simulink model "RedCrane_kinematic_model_joystic"  (R2024a)
settings: Solver=FixedStepAuto  StartTime=0.0  StopTime=inf  FixedStep=Ts  MaxStep=0.005  RelTol=1e-3
values from neighbouring files (symbols this model uses):
  Cartesian_home = [3.55, 0.4, 1.6]'    [enviroment_setup.m]
  M = [1, 0, 0, (L5 + L4 - L1) ... (first row only)    [enviroment_setup.m]
  SList = [ws_mat ... (first row only)    [enviroment_setup.m]
  telescope0 = 0    [enviroment_setup.m]
  thetaList0 = [0, 0,-pi/8, 0, 0]'    [enviroment_setup.m]
  Ts = 0.001    [enviroment_setup.m]
undefined symbols (not defined in the file or in its folder): dp_k_angle_to_stroke, dp_m_angle_to_stroke, p_k_angle_to_stroke, p_k_stroke_to_angle, p_m_angle_to_stroke, p_m_stroke_to_angle, X, Y, Z
libraries: sm_lib x82, nesl_utility x19, fl_lib x16, TcSimInterface x2
(part 1 of 3)
settings Model: Creator=sindr  LastModifiedBy=larso
settings RTWCC: GPUComputeCapability=3.5
settings ConfigComp: PLC_OutputDir=plc_export\FB_JoystickIntegrator  PLC_TargetIDE=twincat3  PLC_MultiTBSigbuilderTimeRange=off  PLC_FoldFBCallOutputVar=off  PLC_RemoveUnusedSSMethodCallArguments=off  PLC_UseCallOutputArgSyntax=off  PLC_EnableUnsignedAndDoubleTypes=off  PLC_EnableUDTSplitting=off  PLC_MaxFieldsInUDT=500  PLC_InlineEnumCastFunction=off

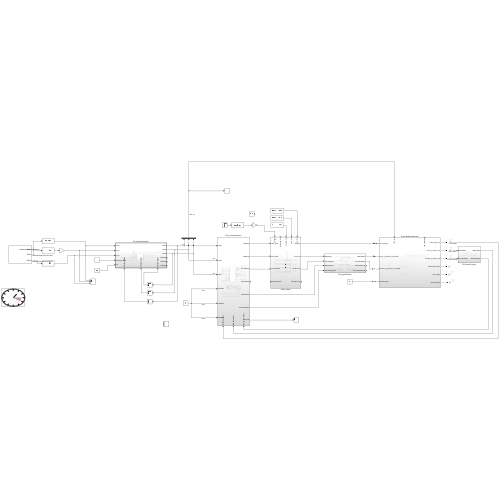
[thumbnail: Simulink's stored preview of the top-level diagram]
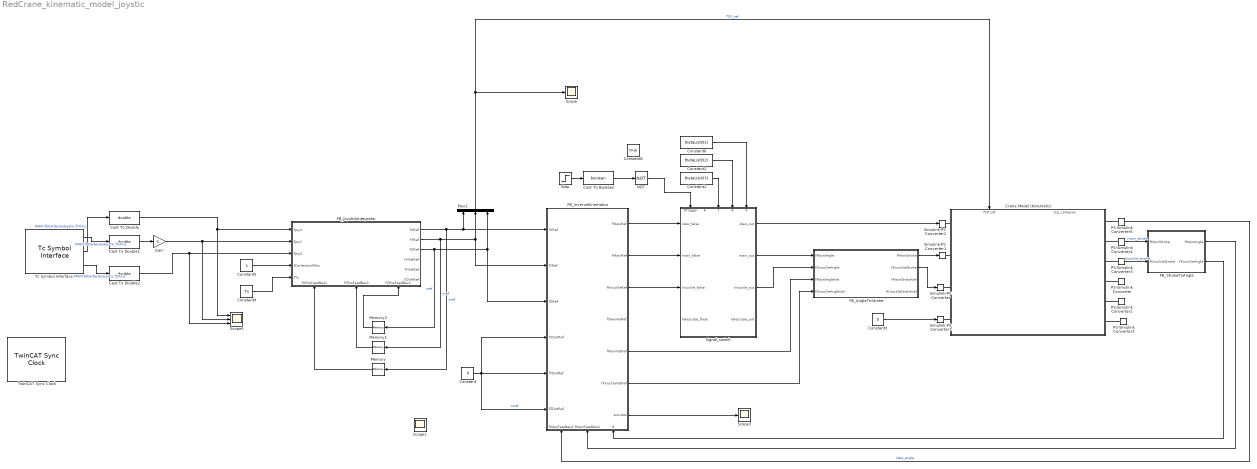
== system RedCrane_kinematic_model_joystic ==
  Cast To Boolean : DataTypeConversion  OutDataTypeStr=boolean  SaturateOnIntegerOverflow=off  RndMeth=Floor
  Cast To Double : DataTypeConversion  OutDataTypeStr=double  SaturateOnIntegerOverflow=off  RndMeth=Floor
  Cast To Double1 : DataTypeConversion  OutDataTypeStr=double  SaturateOnIntegerOverflow=off  RndMeth=Floor
  Cast To Double2 : DataTypeConversion  OutDataTypeStr=double  SaturateOnIntegerOverflow=off  RndMeth=Floor
  Constant : Constant  Value=0
  Constant1 : Constant  Value=thetaList0(3)
  Constant2 : Constant  Value=thetaList0(2)
  Constant3 : Constant  Value=0
  Constant4 : Constant  Value=Ts
  Constant5 : Constant
  Constant6 : Constant  Value=thetaList0(1)
  Constant8 : Constant  Value=true
  Crane Model (Kinematic) : Subsystem
      settings: PortSchema="{\"entries\":[{\"content\":{\"sides\":[{\"content\":{\"connectorIds\":[\"LConn1\",\"LConn2\",\"LConn3\",\"LConn4\"]},\"type\":\"ConnectorPlacement.EquallySpacedRectSide\",\"uuid\":\"4a665765-5f1a-426d-91c2-f3af20fe3627\"},{\"content\":{\"connectorIds\":[\"RConn1\",\"RConn2\",\"RConn3\",\"RConn4\",\"RConn5\",\"RConn6\"],\"side\":\"RIGHT\"},\"type\":\"ConnectorPlacement.EquallySpacedRectSide\",\"uuid\":\"cf43645c-9a50-4bc9-b355-f38e72b1430d\"},{\"content\":{\"connectorIds\":[\"In1\",\"Out1\"],\"side\":\"TOP\"},\"type\":\"ConnectorPlacement.EquallySpacedRectSide\",\"uuid\":\"253dbb23-7a12-4bfe-bf07-7d8403188f09\"}]},\"type\":\"ConnectorPlacement.EquallySpacedConnector\",\"uuid\":\"5ffb1dcc-76b9-4b5c-ba8f-4653fe2f07c9\"}],\"packageUris\":[\"http://schema.mathworks.com/mf0/Connector/R2020b\"],\"version\":\"1.0\"}"
  FB_AngleToStroke : Subsystem
  FB_InverceKinematics : Subsystem
      settings: PortSchema="{\"entries\":[{\"content\":{\"sides\":[{\"content\":{\"connectorIds\":[\"In1\",\"In2\",\"In3\",\"In4\",\"In5\",\"In6\"]},\"type\":\"ConnectorPlacement.EquallySpacedRectSide\",\"uuid\":\"b7f3f39a-cc1b-4519-b948-004466b4d293\"},{\"content\":{\"connectorIds\":[\"Out1\",\"Out2\",\"Out3\",\"Out4\",\"Out5\",\"Out6\",\"Out7\"],\"side\":\"RIGHT\"},\"type\":\"ConnectorPlacement.EquallySpacedRectSide\",\"uuid\":\"cf571c2f-2cc7-4d1d-bbc1-a75d80a0878e\"},{\"content\":{\"side\":\"TOP\"},\"type\":\"ConnectorPlacement.EquallySpacedRectSide\",\"uuid\":\"3f697bd9-7750-4474-8da5-1be48ba53c7e\"},{\"content\":{\"connectorIds\":[\"In7\",\"In8\",\"In9\"],\"side\":\"BOTTOM\"},\"type\":\"ConnectorPlacement.EquallySpacedRectSide\",\"uuid\":\"03fa0a4e-eedb-4a48-8076-446c86a2b4f7\"}]},\"type\":\"ConnectorPlacement.EquallySpacedConnector\",\"uuid\":\"6732c767-80e6-425f-b878-60bd961dd78b\"}],\"packageUris\":[\"http://schema.mathworks.com/mf0/Connector/R2020b\"],\"version\":\"1.0\"}"
  FB_JoystickIntegrator : Subsystem  TreatAsAtomicUnit=on
      settings: PortSchema="{\"entries\":[{\"content\":{\"sides\":[{\"content\":{\"connectorIds\":[\"In1\",\"In2\",\"In3\",\"In4\",\"In5\"]},\"type\":\"ConnectorPlacement.EquallySpacedRectSide\",\"uuid\":\"c5a43198-5d69-4109-b42d-a486a01365c9\"},{\"content\":{\"connectorIds\":[\"Out1\",\"Out2\",\"Out3\",\"Out4\",\"Out5\",\"Out6\"],\"side\":\"RIGHT\"},\"type\":\"ConnectorPlacement.EquallySpacedRectSide\",\"uuid\":\"946526c4-79a3-48b0-aa19-78137d37b9af\"},{\"content\":{\"side\":\"TOP\"},\"type\":\"ConnectorPlacement.EquallySpacedRectSide\",\"uuid\":\"3e7a8b0e-fb34-4723-a326-d25029c5eff4\"},{\"content\":{\"connectorIds\":[\"In6\",\"In7\",\"In8\"],\"side\":\"BOTTOM\"},\"type\":\"ConnectorPlacement.EquallySpacedRectSide\",\"uuid\":\"08712ddf-52dd-443f-9387-c4c8877ba279\"}]},\"type\":\"ConnectorPlacement.EquallySpacedConnector\",\"uuid\":\"e430af44-ed31-458a-a857-840c080c5723\"}],\"packageUris\":[\"http://schema.mathworks.com/mf0/Connector/R2020b\"],\"version\":\"1.0\"}"
  FB_StrokeToAngle : Subsystem
  Gain : Gain  Gain=-1
  Memory : Memory  InitialCondition=Cartesian_home(1)-0.5
  Memory1 : Memory  InitialCondition=Cartesian_home(2)
  Memory2 : Memory  InitialCondition=Cartesian_home(3)
  Mux2 : Mux  Inputs=3
  NOT : Logic  Operator=NOT  IconShape=distinctive  AllPortsSameDT=off  OutDataTypeStr=boolean
  PS-Simulink Converter{,1..5} (6 alike) : nesl_utility/PS-Simulink Converter  PhysicalDomain=network_engine_domain  SubClassName=ps_output  LeftPortType=input  RightPortType=output  PseudoPeriodic=off  Frequencies=[]  VectorFormat=inherit  Unit=inherit  AffineConversion=off
  Scope : Scope
  Scope1 : Scope  NumInputPorts=3
  Scope3 : Scope
  Scope5 : Scope  NumInputPorts=3
  Signal_switch : Subsystem
      settings: PortSchema="{\"entries\":[{\"content\":{\"sides\":[{\"content\":{\"connectorIds\":[\"In1\",\"In2\",\"In3\",\"In4\"]},\"type\":\"ConnectorPlacement.EquallySpacedRectSide\",\"uuid\":\"677999b9-dfe1-4592-affa-fb9b7d257ea0\"},{\"content\":{\"connectorIds\":[\"Out1\",\"Out2\",\"Out3\",\"Out4\"],\"side\":\"RIGHT\"},\"type\":\"ConnectorPlacement.EquallySpacedRectSide\",\"uuid\":\"3f36c443-9717-41bf-801d-3d95a9d66f59\"},{\"content\":{\"connectorIds\":[\"In5\",\"In6\",\"In7\",\"In8\",\"In9\"],\"side\":\"TOP\"},\"type\":\"ConnectorPlacement.EquallySpacedRectSide\",\"uuid\":\"b7ea9b48-8dcd-4abb-ae26-aa1832701a6a\"}]},\"type\":\"ConnectorPlacement.EquallySpacedConnector\",\"uuid\":\"7d55d43f-82cc-482c-a650-cc44ad6cee22\"}],\"packageUris\":[\"http://schema.mathworks.com/mf0/Connector/R2020b\"],\"version\":\"1.0\"}"
  Simulink-PS Converter{,1..3} (4 alike) : nesl_utility/Simulink-PS Converter  PhysicalDomain=network_engine_domain  SubClassName=ps_input  LeftPortType=input  RightPortType=output  PseudoPeriodic=off  Frequencies=[]  NoiseDistribution=none  NoiseParameters=[]  Unit=1  AffineConversion=off  FilteringAndDerivatives=filter  SimscapeFilterOrder=2  InputFilterTimeConstant=0.001  UdotUserProvided=0
  Step : Step  SampleTime=0
  Tc Symbol Interface1 : TcSimInterface/Tc Symbol Interface  ChangeRowColOrder=on  TraceMode=3  DirectFeedThrough=0  SignalLabels=3  PortLabels=2  ExpandBusObjDepth=on  RuntimeConfig=|  SymbolInterfaceInfo=|  SyncClockMode=1
      RuntimeConfig=|
      | <?xml version="1.0" encoding="UTF-8" standalone="no"?>
      | <TcRuntimAdapterProject>
      | 	<DataTypes>
      | 		<DataType>
      | 			<Name GUID="{3BC82419-4CB4-48F5-8384-E3D86DEA2DAE}" Namespace="TcDataExchange">ITcStreamAdsRequestHandler</Name>
      | 			<BitSize X64="64">32</BitSize>
      | 			<BaseType GUID="{00000001-0000-0000-E000-000000000064}">ITcUnknown</BaseType>
      | 			<Method>
      | 				<Name>Send</Name>
      | 				<ReturnType GUID="{18071995-0000-0000-0000-000000000019}">HRESULT</ReturnType>
      | 				<ReturnBitSize>32</ReturnBitSize>
      | 				<Parameter>
      | 					<Name>timeoutMs</Name>
      | 					<Type GUID="{18071995-0000-0000-0000-000000000006}" Optional="1000">INT</Type>
      | 					<BitSize>16</BitSize>
      | 				</Parameter>
      | 				<Parameter>
      | 					<Name>timeStamp</Name>
      | 					<Type GUID="{18071995-0000-0000-0000-00000000000C}" Optional="0">LINT</Type>
      | 					<BitSize>64</BitSize>
      | 				</Parameter>
      | 			</Method>
      | 			<Method>
      | 				<Name>GetResult</Name>
      | 				<ReturnType GUID="{18071995-0000-0000-0000-000000000019}">HRESULT</ReturnType>
      | 				<ReturnBitSize>32</ReturnBitSize>
      | 				<Parameter>
      | 					<Name>pErrorCode</Name>
      | 					<Type GUID="{18071995-0000-0000-0000-000000000009}" PointerTo="1" RpcDirection="out">DINT</Type>
      | 					<BitSize X64="64">32</BitSize>
      | 				</Parameter>
      | 				<Parameter>
      | 					<Name>wait</Name>
      | 					<Type GUID="{18071995-0000-0000-0000-000000000030}" Optional="0">BOOL</Type>
      | 					<BitSize>8</BitSize>
      | 				</Parameter>
      | 			</Method>
      | 			<Method>
      | 				<Name>Cancel</Name>
      | 				<ReturnType GUID="{18071995-0000-0000-0000-000000000019}">HRESULT</ReturnType>
      | 				<ReturnBitSize>32</ReturnBitSize>
      | 			</Method>
      | 			<Hides>
      | 				<Hide GUID="{D5D4EABE-5709-4F1D-A52D-DD780CF3BEE8}"/>
      | 				<Hide GUID="{96230612-048D-4927-9A3E-E69B743416F7}"/>
      | 				<Hide GUID="{F0F623C7-A650-457C-A27C-87DC2B08989E}"/>
      | 				<Hide GUID="{18FCA6B6-AFA6-45DD-BC02-F3037EA03FB7}"/>
      | 				<Hide GUID="{12AC5FFF-B3F6-4F3E-8EDD-8044D44F084F}"/>
      | 				<Hide GUID="{6CDF8435-1307-4137-94DE-D793A77839C3}"/>
      | 				<Hide GUID="{D7B34C9A-90C5-4E79-A290-017678319005}"/>
      | 			</Hides>
      | 		</DataType>
      | 		<DataType>
      | 			<Name GUID="{18071995-0000-0000-0000-000000000041}" TcBaseType="true" HideSubItems="true" CName="AmsNetId">AMSNETID</Name>
      | 			<BitSize>48</BitSize>
      | 			<BaseType GUID="{18071995-0000-0000-0000-000000000001}">BYTE</BaseType>
      | 			<ArrayInfo>
      | 				<LBound>0</LBound>
      | 				<Elements>6</Elements>
      | 			</ArrayInfo>
      | 			<Format>
      | 				<Printf>%d.%d.%d.%d.%d.%d</Printf>
      | 				<Parameter>[0]</Parameter>
      | 				<Parameter>[1]</Parameter>
      | 				<Parameter>[2]</Parameter>
      | 				<Parameter>[3]</Parameter>
      | 				<Parameter>[4]</Parameter>
      | 				<Parameter>[5]</Parameter>
      | 			</Format>
      | 		</DataType>
      | 		<DataType>
      | 			<Name GUID="{18071995-0000-0000-0000-000000000042}" TcBaseType="true" CName="AmsAddr">AMSADDR</Name>
      | 			<BitSize>64</BitSize>
      | 			<SubItem>
      | 				<Name>netId</Name>
      | 				<Type GUID="{18071995-0000-0000-0000-000000000041}">AMSNETID</Type>
      | 				<BitSize>48</BitSize>
      | 				<BitOffs>0</BitOffs>
      | 			</SubItem>
      | 			<SubItem>
      | 				<Name>port</Name>
      | 				<Type GUID="{18071995-0000-0000-0000-000000000004}">WORD</Type>
      | 				<BitSize>16</BitSize>
      | 				<BitOffs>48</BitOffs>
      | 			</SubItem>
      | 			<Format>
      | 				<Printf>%d.%d.%d.%d.%d.%d:%d</Printf>
      | 				<Parameter>.netId[0]</Parameter>
      | 				<Parameter>.netId[1]</Parameter>
      | 				<Parameter>.netId[2]</Parameter>
      | 				<Parameter>.netId[3]</Parameter>
      | 				<Parameter>.netId[4]</Parameter>
      | 				<Parameter>.netId[5]</Parameter>
      | 				<Parameter>.port</Parameter>
      | 			</Format>
      | 			<Format Name="Iec">
      | 				<Printf>(netId:=[%d.%d.%d.%d.%d.%d], port :=%d)</Printf>
      | 				<Parameter>.netId[0]</Parameter>
      | 				<Parameter>.netId[1]</Parameter>
      | 				<Parameter>.netId[2]</Parameter>
      | 				<Parameter>.netId[3]</Parameter>
      | 				<Parameter>.netId[4]</Parameter>
      | 				<Parameter>.netId[5]</Parameter>
      | 				<Parameter>.port</Parameter>
      | 			</Format>
      | 		</DataType>
      | 		<DataType>
      | 			<Name GUID="{EA8975F7-A358-4090-8A68-57EC94D47710}" Namespace="TcDataExchange">SampleCopyInfo</Name>
      | 			<BitSize X64="192">160</BitSize>
      | 			<SubItem>
      | 				<Name>PData</Name>
      | 				<Type GUID="{18071995-0000-0000-0000-000000000001}" PointerTo="1">BYTE</Type>
      | 				<BitSize X64="64">32</BitSize>
      | 				<BitOffs>0</BitOffs>
      | 			</SubItem>
      | 			<SubItem>
      | 				<Name>CbData</Name>
      | 				<Type GUID="{18071995-0000-0000-0000-000000000008}">UDINT</Type>
      | 				<BitSize>32</BitSize>
      | 				<BitOffs X64="64">32</BitOffs>
      | 			</SubItem>
      | 			<SubItem>
      | 				<Name>ErrorCode</Name>
      | 				<Type GUID="{18071995-0000-0000-0000-000000000009}">DINT</Type>
      | 				<BitSize>32</BitSize>
      | 				<BitOffs X64="96">64</BitOffs>
      | 			</SubItem>
      | 			<SubItem>
      | 				<Name>Timestamp</Name>
      | 				<Type GUID="{18071995-0000-0000-0000-00000000000C}">LINT</Type>
      | 				<BitSize>64</BitSize>
      | 				<BitOffs X64="128">96</BitOffs>
      | 			</SubItem>
      | 			<Hides>
      | 				<Hide GUID="{97351DCE-1E32-4BD2-BF27-53E71AD5C45D}"/>
      | 				<Hide GUID="{ED3F58EE-1A95-40F4-94DA-D825E6682038}"/>
      | 				<Hide GUID="{82197966-3CEC-4E84-8982-F64641125942}"/>
      | 			</Hides>
      | 		</DataType>
      | 		<DataType>
      | 			<Name GUID="{9165C8A1-78D1-4B81-89D0-BA48F61AF93B}" Namespace="TcDataExchange">ITcStreamSynchronizer</Name>
      | 			<Comment TxtId=""><![CDATA[Provides time synchronisation between data sources and data sinks in different time contexts. A time context might be a real time TwinCAT system the simulation time of a simulation tool or the basic time stamp of logged data in a database.]]></Comment>
      | 			<BitSize X64="64">32</BitSize>
      | 			<BaseType GUID="{00000001-0000-0000-E000-000000000064}">ITcUnknown</BaseType>
      | 			<Method>
      | 				<Name>RegisterTimeContext</Name>
      | 				<Comment><![CDATA[Registers a time context for synchronization. Registration has to be completet for all time contexts before starting the communication. ]]></Comment>
      | 				<ReturnType GUID="{18071995-0000-0000-0000-000000000019}">HRESULT</ReturnType>
      | 				<ReturnBitSize>32</ReturnBitSize>
      | 				<Parameter>
      | 					<Name>pSyncId</Name>
      | 					<Comment><![CDATA[Unique identifier of the time context. This might be e.g. the AmsNetId of a TwinCAT system or a ULINT representation of a logged dataset.]]></Comment>
      | 					<Type GUID="{18071995-0000-0000-0000-000000000021}" PointerTo="1">GUID</Type>
      | 					<BitSize X64="64">32</BitSize>
      | 				</Parameter>
      | 				<Parameter>
      | 					<Name>timeStamp</Name>
      | 					<Comment><![CDATA[Timestamp of the first received sample]]></Comment>
      | 					<Type GUID="{18071995-0000-0000-0000-00000000000C}">LINT</Type>
      | 					<BitSize>64</BitSize>
      | 				</Parameter>
      | 			</Method>
      | 			<Method>
      | 				<Name>TransformTime</Name>
      | 				<ReturnType GUID="{18071995-0000-0000-0000-000000000019}">HRESULT</ReturnType>
      | 				<ReturnBitSize>32</ReturnBitSize>
      | 				<Parameter>
      | 					<Name>pSourceSyncId</Name>
      | 					<Comment><![CDATA[Unique identifier of the source time context.]]></Comment>
      | 					<Type GUID="{18071995-0000-0000-0000-000000000021}" PointerTo="1">GUID</Type>
      | 					<BitSize X64="64">32</BitSize>
      | 				</Parameter>
      | 				<Parameter>
      | 					<Name>pSinkSyncId</Name>
      | 					<Comment><![CDATA[Unique identifier of the sink time context.]]></Comment>
      | 					<Type GUID="{18071995-0000-0000-0000-000000000021}" PointerTo="1">GUID</Type>
      | 					<BitSize X64="64">32</BitSize>
      | 				</Parameter>
      | 				<Parameter>
      | 					<Name>timeStamp</Name>
      | 					<Comment><![CDATA[Expects the sink timestamp and returns the appropriate source timestamp.
      | If the specified sink sync ID is unknown, the sink timestamp is register as its start time.]]></Comment>
      | 					<Type GUID="{18071995-0000-0000-0000-00000000000C}" ReferenceTo="true">LINT</Type>
      | 					<BitSize X64="64">32</BitSize>
      | 				</Parameter>
      | 			</Method>
      | 			<Hides>
      | 				<Hide GUID="{92EEAEA2-3DA4-48E7-A741-8C78A0326B08}"/>
      | 				<Hide GUID="{4F229E80-CBB0-4042-863E-770932FFF733}"/>
      | 				<Hide GUID="{BDB7FF6F-6144-4421-92B4-18BEEF6031E5}"/>
      | 				<Hide GUID="{5983EBFA-553B-4573-BA8B-8294D34A7664}"/>
      | 				<Hide GUID="{8DB2BF24-3BB5-46A0-91E8-A1C18BBD84A4}"/>
      | 				<Hide GUID="{865BE9CA-A112-4D69-9BA4-637F3C45508E}"/>
      | 				<Hide GUID="{5732FA65-993E-4C75-A424-0F55737580DD}"/>
      | 				<Hide GUID="{E7473B34-EFDE-47D8-AEF4-4BDF09E5E870}"/>
      | 				<Hide GUID="{BA2BDE8E-989A-4914-98EA-E301FA5E0803}"/>
      | 				<Hide GUID="{59CDFCE5-FBBF-47C8-A338-68414C56327E}"/>
      | 				<Hide GUID="{0C52276D-0720-4AEF-8258-67851E35C9C8}"/>
      | 				<Hide GUID="{4A5DD8C7-96C5-4D47-A240-8E493B9287A7}"/>
      | 			</Hides>
      | 		</DataType>
      | 		<DataType>
      | 			<Name GUID="{CD026BE9-DD1E-4238-B09F-CDE426934EFB}" Namespace="TcDataExchange">ITcStreamSyncDataSink</Name>
      | 			<BitSize X64="64">32</BitSize>
      | 			<BaseType GUID="{00000001-0000-0000-E000-000000000064}">ITcUnknown</BaseType>
      | 			<Method>
      | 				<Name>WriteSamples</Name>
      | 				<ReturnType GUID="{18071995-0000-0000-0000-000000000019}">HRESULT</ReturnType>
      | 				<ReturnBitSize>32</ReturnBitSize>
      | 				<Parameter>
      | 					<Name>writerOid</Name>
      | 					<Type GUID="{18071995-0000-0000-0000-00000000000F}">OTCID</Type>
      | 					<BitSize>32</BitSize>
      | 				</Parameter>
      | 				<Parameter>
      | 					<Name>pSyncId</Name>
      | 					<Comment><![CDATA[Unique identifier of the time context. This might be e.g. the AmsNetId of a TwinCAT system or a ULINT representation of a logged dataset.]]></Comment>
      | 					<Type GUID="{18071995-0000-0000-0000-000000000021}" PointerTo="1" RpcDirection="in">GUID</Type>
      | 					<BitSize X64="64">32</BitSize>
      | 				</Parameter>
      | 				<Parameter>
      | 					<Name>sampleSize</Name>
      | 					<Type GUID="{18071995-0000-0000-0000-000000000008}" RpcDirection="in">UDINT</Type>
      | 					<BitSize>32</BitSize>
      | 				</Parameter>
      | 				<Parameter>
      | 					<Name>sampleCount</Name>
      | 					<Type GUID="{18071995-0000-0000-0000-000000000008}" RpcDirection="in">UDINT</Type>
      | 					<BitSize>32</BitSize>
      | 				</Parameter>
      | 				<Parameter>
      | 					<Name>pSamples</Name>
      | 					<Type GUID="{18071995-0000-0000-0000-000000000001}" PointerTo="1" RpcDirection="in">BYTE</Type>
      | 					<BitSize X64="64">32</BitSize>
      | 				</Parameter>
      | 				<Parameter>
      | 					<Name>pErrorCodes</Name>
      | 					<Type GUID="{18071995-0000-0000-0000-000000000009}" PointerTo="1" RpcDirection="in" RpcLengthIs="sampleCount" Optional="0">DINT</Type>
      | 					<BitSize X64="64">32</BitSize>
      | 				</Parameter>
      | 				<Parameter>
      | 					<Name>pTimeStamps</Name>
      | 					<Type GUID="{18071995-0000-0000-0000-00000000000C}" PointerTo="1" RpcDirection="in" Optional="0">LINT</Type>
      | 					<BitSize X64="64">32</BitSize>
      | 				</Parameter>
      | 				<Parameter>
      | 					<Name>sampleStride</Name>
      | 					<Type GUID="{18071995-0000-0000-0000-000000000006}" Optional="-1">INT</Type>
      | 					<BitSize>16</BitSize>
      | 				</Parameter>
      | 				<Parameter>
      | 					<Name>errorCodeStride</Name>
      | 					<Type GUID="{18071995-0000-0000-0000-000000000006}" Optional="-1">INT</Type>
      | 					<BitSize>16</BitSize>
      | 				</Parameter>
      | 				<Parameter>
      | 					<Name>timeStampStride</Name>
      | 					<Type GUID="{18071995-0000-0000-0000-000000000006}" Optional="-1">INT</Type>
      | 					<BitSize>16</BitSize>
      | 				</Parameter>
      | 			</Method>
      | 			<Method>
      | 				<Name>WriteSamples</Name>
      | 				<ReturnType GUID="{18071995-0000-0000-0000-000000000019}">HRESULT</ReturnType>
      | 				<ReturnBitSize>32</ReturnBitSize>
      | 				<Parameter>
      | 					<Name>pSyncId</Name>
      | 					<Comment><![CDATA[Unique identifier of the time context. This might be e.g. the AmsNetId of a TwinCAT system or a ULINT representation of a logged dataset.]]></Comment>
      | 					<Type GUID="{18071995-0000-0000-0000-000000000021}" PointerTo="1" RpcDirection="in">GUID</Type>
      | 					<BitSize X64="64">32</BitSize>
      | 				</Parameter>
      | 				<Parameter>
      | 					<Name>sampleCount</Name>
      | 					<Type GUID="{18071995-0000-0000-0000-000000000008}" RpcDirection="in">UDINT</Type>
      | 					<BitSize>32</BitSize>
      | 				</Parameter>
      | 				<Parameter>
      | 					<Name>pSampleCopyInfo</Name>
      | 					<Type GUID="{EA8975F7-A358-4090-8A68-57EC94D47710}" Namespace="TcDataExchange" PointerTo="1" RpcDirection="in">SampleCopyInfo</Type>
      | 					<BitSize X64="64">32</BitSize>
      | 				</Parameter>
      | 			</Method>
      | 			<Method>
      | 				<Name>GetSynchronizer</Name>
      | 				<ReturnType GUID="{18071995-0000-0000-0000-000000000019}">HRESULT</ReturnType>
      | 				<ReturnBitSize>32</ReturnBitSize>
      | 				<Parameter>
      | 					<Name>ppSynchronizer</Name>
      | 					<Type GUID="{9165C8A1-78D1-4B81-89D0-BA48F61AF93B}" Namespace="TcDataExchange" PointerTo="1">ITcStreamSynchronizer</Type>
      | 					<BitSize X64="64">32</BitSize>
      | 				</Parameter>
      | 			</Method>
      | 			<Hides>
      | 				<Hide GUID="{81DCA55F-6320-4831-9AAA-FA43AB137432}"/>
      | 				<Hide GUID="{7F649ADE-4559-4067-8B4B-52A9AFF9D566}"/>
      | 				<Hide GUID="{1ACFD07C-85DE-4584-B8DF-DCE4B2186A56}"/>
      | 				<Hide GUID="{001A190B-B452-4F64-99FE-587E5CB0E1C9}"/>
      | 				<Hide GUID="{D321BA65-82B7-4E6F-9E21-63A2CF6BE6E4}"/>
      | 				<Hide GUID="{59469964-9185-47B0-8E1F-A41A5243C9A7}"/>
      | 				<Hide GUID="{50E978C6-91D0-425B-941B-FF6E10C52E19}"/>
      | 				<Hide GUID="{2B2E9620-3973-41C2-927F-D2660E0236D6}"/>
      | 				<Hide GUID="{4C925035-5840-4BD6-BA08-B62ECBE72975}"/>
      | 				<Hide GUID="{C77882D3-FF3C-4E62-96AB-AB67CC7FA3B0}"/>
      | 				<Hide GUID="{7619FBA7-E9CC-47D7-AEE2-2BAE64602CA0}"/>
      | 				<Hide GUID="{CACC088B-451D-4181-939C-F28316D26AF6}"/>
      | 				<Hide GUID="{1701C290-46E1-4294-AA28-C9384682A3D1}"/>
      | 				<Hide GUID="{D4FE94A8-2959-45FC-B97D-A36FE755F217}"/>
      | 				<Hide GUID="{62A55225-FD8F-4450-A003-5E82394FD0D1}"/>
      | 				<Hide GUID="{7DA0071B-E1EB-4FCF-B5BE-180B5FA4841C}"/>
      | 				<Hide GUID="{D2B3A2BF-4D63-4F61-853F-3333868D1C42}"/>
      | 				<Hide GUID="{C8B9397B-AE09-4B06-8883-D01BD9BBDEFB}"/>
      | 				<Hide GUID="{276A390F-8541-45D2-8A94-8E3B6B609E81}"/>
      | 				<Hide GUID="{F4C49966-BC54-424E-A3C6-69D9FBDDE2BC}"/>
      | 			</Hides>
      | 		</DataType>
      | 		<DataType>
      | 			<Name GUID="{877CB26F-4EC1-469B-9F87-706DDBDA821F}" Namespace="TcDataExchange">ITcStreamSyncDataSource</Name>
      | 			<BitSize X64="64">32</BitSize>
      | 			<BaseType GUID="{00000001-0000-0000-E000-000000000064}">ITcUnknown</BaseType>
      | 			<Method>
      | 				<Name>ReadSamples</Name>
      | 				<ReturnType GUID="{18071995-0000-0000-0000-000000000019}">HRESULT</ReturnType>
      | 				<ReturnBitSize>32</ReturnBitSize>
      | 				<Parameter>
      | 					<Name>readerOid</Name>
      | 					<Type GUID="{18071995-0000-0000-0000-00000000000F}">OTCID</Type>
      | 					<BitSize>32</BitSize>
      | 				</Parameter>
      | 				<Parameter>
      | 					<Name>pSyncId</Name>
      | 					<Comment><![CDATA[Unique identifier of the time context. This might be e.g. the AmsNetId of a TwinCAT system or a ULINT representation of a logged dataset.]]></Comment>
      | 					<Type GUID="{18071995-0000-0000-0000-000000000021}" PointerTo="1" RpcDirection="in">GUID</Type>
      | 					<BitSize X64="64">32</BitSize>
      | 				</Parameter>
      | 				<Parameter>
      | 					<Name>sampleSize</Name>
      | 					<Type GUID="{18071995-0000-0000-0000-000000000008}" RpcDirection="in">UDINT</Type>
      | 					<BitSize>32</BitSize>
      | 				</Parameter>
      | 				<Parameter>
      | 					<Name>sampleCount</Name>
      | 					<Type GUID="{18071995-0000-0000-0000-000000000008}" ReferenceTo="true" RpcDirection="in">UDINT</Type>
      | 					<BitSize X64="64">32</BitSize>
      | 				</Parameter>
      | 				<Parameter>
      | 					<Name>pSamples</Name>
      | 					<Type GUID="{18071995-0000-0000-0000-000000000001}" PointerTo="1" RpcDirection="out">BYTE</Type>
      | 					<BitSize X64="64">32</BitSize>
      | 				</Parameter>
      | 				<Parameter>
      | 					<Name>pErrorCodes</Name>
      | 					<Type GUID="{18071995-0000-0000-0000-000000000009}" PointerTo="1" RpcDirection="out" RpcLengthIs="sampleCount" Optional="0">DINT</Type>
      | 					<BitSize X64="64">32</BitSize>
      | 				</Parameter>
      | 				<Parameter>
      | 					<Name>pTimeStamps</Name>
      | 					<Type GUID="{18071995-0000-0000-0000-00000000000C}" PointerTo="1" RpcDirection="out" RpcLengthIs="sampleCount" Optional="0">LINT</Type>
      | 					<BitSize X64="64">32</BitSize>
      | 				</Parameter>
      | 				<Parameter>
      | 					<Name>timeStamp</Name>
      | 					<Type GUID="{18071995-0000-0000-0000-00000000000C}" Optional="0">LINT</Type>
      | 					<BitSize>64</BitSize>
      | 				</Parameter>
      | 				<Parameter>
      | 					<Name>nextTimeStamp</Name>
      | 					<Type GUID="{18071995-0000-0000-0000-00000000000C}" Optional="0">LINT</Type>
      | 					<BitSize>64</BitSize>
      | 				</Parameter>
      | 			</Method>
      | 			<Method>
      | 				<Name>ReadSamples</Name>
      | 				<ReturnType GUID="{18071995-0000-0000-0000-000000000019}">HRESULT</ReturnType>
      | 				<ReturnBitSize>32</ReturnBitSize>
      | 				<Parameter>
      | 					<Name>readerOid</Name>
      | 					<Type GUID="{18071995-0000-0000-0000-00000000000F}">OTCID</Type>
      | 					<BitSize>32</BitSize>
      | 				</Parameter>
      | 				<Parameter>
      | 					<Name>pSyncId</Name>
      | 					<Comment><![CDATA[Unique identifier of the time context. This might be e.g. the AmsNetId of a TwinCAT system or a ULINT representation of a logged dataset.]]></Comment>
      | 					<Type GUID="{18071995-0000-0000-0000-000000000021}" PointerTo="1" RpcDirection="in">GUID</Type>
      | 					<BitSize X64="64">32</BitSize>
      | 				</Parameter>
      | 				<Parameter>
      | 					<Name>sampleCount</Name>
      | 					<Type GUID="{18071995-0000-0000-0000-000000000008}" ReferenceTo="true" RpcDirection="in">UDINT</Type>
      | 					<BitSize X64="64">32</BitSize>
      | 				</Parameter>
      | 				<Parameter>
      | 					<Name>pSampleCopyInfo</Name>
      | 					<Type GUID="{EA8975F7-A358-4090-8A68-57EC94D47710}" Namespace="TcDataExchange" PointerTo="1" RpcLengthIs="sampleCount">SampleCopyInfo</Type>
      | 					<BitSize X64="64">32</BitSize>
      | 				</Parameter>
      | 				<Parameter>
      | 					<Name>timeStamp</Name>
      | 					<Type GUID="{18071995-0000-0000-0000-00000000000C}" Optional="0">LINT</Type>
      | 					<BitSize>64</BitSize>
      | 				</Parameter>
      | 				<Parameter>
      | 					<Name>nextTimeStamp</Name>
      | 					<Type GUID="{18071995-0000-0000-0000-00000000000C}" Optional="0">LINT</Type>
      | 					<BitSize>64</BitSize>
      | 				</Parameter>
      | 			</Method>
      | 			<Method>
      | 				<Name>ReadSample</Name>
      | 				<ReturnType GUID="{18071995-0000-0000-0000-000000000019}">HRESULT</ReturnType>
      | 				<ReturnBitSize>32</ReturnBitSize>
      | 				<Parameter>
      | 					<Name>readerOid</Name>
      | 					<Type GUID="{18071995-0000-0000-0000-00000000000F}">OTCID</Type>
      | 					<BitSize>32</BitSize>
      | 				</Parameter>
      | 				<Parameter>
      | 					<Name>pSyncId</Name>
      | 					<Comment><![CDATA[Unique identifier of the time context. This might be e.g. the AmsNetId of a TwinCAT system or a ULINT representation of a logged dataset.]]></Comment>
      | 					<Type GUID="{18071995-0000-0000-0000-000000000021}" PointerTo="1" RpcDirection="in">GUID</Type>
      | 					<BitSize X64="64">32</BitSize>
      | 				</Parameter>
      | 				<Parameter>
      | 					<Name>sampleSize</Name>
      | 					<Type GUID="{18071995-0000-0000-0000-000000000008}" RpcDirection="in">UDINT</Type>
      | 					<BitSize>32</BitSize>
      | 				</Parameter>
      | 				<Parameter>
      | 					<Name>timeStamp</Name>
      | 					<Type GUID="{18071995-0000-0000-0000-00000000000C}" RpcDirection="in">LINT</Type>
      | 					<BitSize>64</BitSize>
      | 				</Parameter>
      | 				<Parameter>
      | 					<Name>pSample</Name>
      | 					<Type GUID="{18071995-0000-0000-0000-000000000001}" PointerTo="1" RpcDirection="out">BYTE</Type>
      | 					<BitSize X64="64">32</BitSize>
      | 				</Parameter>
      | 				<Parameter>
      | 					<Name>nextTimeStamp</Name>
      | 					<Type GUID="{18071995-0000-0000-0000-00000000000C}" Optional="0">LINT</Type>
      | 					<BitSize>64</BitSize>
      | 				</Parameter>
      | 				<Parameter>
      | 					<Name>timeoutMs</Name>
      | 					<Type GUID="{18071995-0000-0000-0000-000000000006}" Optional="0">INT</Type>
      | 					<BitSize>16</BitSize>
      | 				</Parameter>
      | 			</Method>
      | 			<Method>
      | 				<Name>ReportTransferState</Name>
      | 				<ReturnType GUID="{18071995-0000-0000-0000-000000000019}">HRESULT</ReturnType>
      | 				<ReturnBitSize>32</ReturnBitSize>
      | 				<Parameter>
      | 					<Name>sampleCount</Name>
      | 					<Type GUID="{18071995-0000-0000-0000-000000000008}" RpcDirection="in">UDINT</Type>
      | 					<BitSize>32</BitSize>
      | 				</Parameter>
      | 				<Parameter>
      | 					<Name>pTimeStamps</Name>
      | 					<Type GUID="{18071995-0000-0000-0000-00000000000B}" PointerTo="1" RpcDirection="in" RpcLengthIs="sampleCount">ULINT</Type>
      | 					<BitSize X64="64">32</BitSize>
      | 				</Parameter>
      | 				<Parameter>
      | 					<Name>pErrorCodes</Name>
      | 					<Type GUID="{18071995-0000-0000-0000-000000000009}" PointerTo="1" RpcDirection="in" RpcLengthIs="sampleCount">DINT</Type>
      | 					<BitSize X64="64">32</BitSize>
      | 				</Parameter>
      | 			</Method>
      | 			<Hides>
      | 				<Hide GUID="{82F08223-5E24-40E3-9A21-D5759118CBB7}"/>
      | 				<Hide GUID="{BC021C3C-19AB-41D1-A0EC-9FBFBB8814F1}"/>
      | 				<Hide GUID="{50FC6FF1-2968-4C30-A0C6-937238137C4E}"/>
      | 				<Hide GUID="{728E78FA-EADA-4107-BAE9-D37F8F7B9F91}"/>
      | 				<Hide GUID="{C24D9FA7-A6FF-412B-8385-D45B3613DB25}"/>
      | 				<Hide GUID="{57723EE7-8620-4304-9DD4-46EA4C8A93FC}"/>
      | 				<Hide GUID="{F29D82E8-B39D-4DDA-9326-A3CDC9CBBA4B}"/>
      | 				<Hide GUID="{53ABEA21-7053-4CE3-9300-41FAB67AF005}"/>
      | 				<Hide GUID="{E5414156-6DAA-44BD-9EFA-B9044BBB9FAE}"/>
      | 				<Hide GUID="{160EC4BE-B114-439C-A4F5-197C13AE54BE}"/>
      | 				<Hide GUID="{D7DC26B1-9810-47CC-88D8-D4B09543C26B}"/>
      | 				<Hide GUID="{2F3D2A75-7CFD-4B59-86BD-5AB92BFF5C6C}"/>
      | 				<Hide GUID="{205321E8-A331-4955-8C9E-2D60B6EAF5D8}"/>
      | 				<Hide GUID="{BA3232D2-3C23-413B-A027-D772D0C5AA3E}"/>
      | 				<Hide GUID="{FAF64FB6-67DC-4FA2-8863-A3D939045635}"/>
      | 				<Hide GUID="{5DF157ED-EE29-443B-ACD3-F7E4A686CAC8}"/>
      | 				<Hide GUID="{E20D9512-3189-4583-A5D1-6C522392AD43}"/>
      | 				<Hide GUID="{F98C9E94-47EC-40AD-AC60-E0D0FB029194}"/>
      | 				<Hide GUID="{4ED484EC-9FA9-4567-9D83-41D6BB37A214}"/>
      | 				<Hide GUID="{48244BB5-38E0-4EC3-BEA8-67AE38BFA0E5}"/>
      | 				<Hide GUID="{D85B01E0-4969-4DCF-BE5B-BBCBD9E96328}"/>
      | 				<Hide GUID="{DF45952D-9A36-4D45-934F-003F97EE2709}"/>
      | 				<Hide GUID="{582175E1-C08A-4DA1-8055-83DB0709413E}"/>
      | 				<Hide GUID="{292D2B8D-7D29-4791-A738-0FA706E6D7C7}"/>
      | 				<Hide GUID="{9660BF40-2F53-4366-912D-5DA5488BD995}"/>
      | 				<Hide GUID="{AA37253E-123B-4A23-88B2-320766B046C5}"/>
      | 				<Hide GUID="{8A9F48A1-52FB-47FA-AF47-A72CB42C8F27}"/>
      | 				<Hide GUID="{DC5918CB-E382-4038-B2ED-00FF581EA40F}"/>
      | 				<Hide GUID="{754FA08E-4EE5-4772-B861-C4D9514E5FE2}"/>
      | 				<Hide GUID="{2C0F86D1-13AC-46DB-BFB0-A62CF0B8CEE8}"/>
      | 			</Hides>
      | 		</DataType>
      | 		<DataType>
      | 			<Name GUID="{2919D6B4-47C4-4AE8-B706-E94C497ECB99}" Namespace="TcDataExchange">NotificationTransMode</Name>
      | 			<BitSize>16</BitSize>
      | 			<BaseType GUID="{18071995-0000-0000-0000-000000000006}">INT</BaseType>
      | 			<EnumInfo>
      | 				<Text><![CDATA[NoTrans]]></Text>
      | 				<Enum>0</Enum>
      | 			</EnumInfo>
      | 			<EnumInfo>
      | 				<Text><![CDATA[ServerCycle]]></Text>
      | 				<Enum>3</Enum>
      | 			</EnumInfo>
      | 			<EnumInfo>
      | 				<Text><![CDATA[OnChange]]></Text>
      | 				<Enum>4</Enum>
      | 			</EnumInfo>
      | 			<Hides>
      | 				<Hide GUID="{79465139-46B4-43EB-B7FF-967BF64C3367}"/>
      | 				<Hide GUID="{AE2F4BB5-B98E-4C79-AC26-086A9CF7EAC6}"/>
      | 				<Hide GUID="{ECF929B2-79C7-483F-A3DC-06B91AFD531C}"/>
      | 				<Hide GUID="{4E4B27B2-E550-42F1-92B6-1EFABDB0481B}"/>
      | 			</Hides>
      | 		</DataType>
      | 		<DataType>
      | 			<Name GUID="{B75DDCED-7BC8-45F5-8D80-27345642612D}" Namespace="TcDataExchange">NotificationState</Name>
      | 			<BitSize>16</BitSize>
      | 			<BaseType GUID="{18071995-0000-0000-0000-000000000006}">INT</BaseType>
      | 			<EnumInfo>
      | 				<Text><![CDATA[Stop]]></Text>
      | 				<Enum>0</Enum>
      | 			</EnumInfo>
      | 			<EnumInfo>
      | 				<Text><![CDATA[Starting]]></Text>
      | 				<Enum>1</Enum>
      | 			</EnumInfo>
      | 			<EnumInfo>
      | 				<Text><![CDATA[Run]]></Text>
      | 				<Enum>2</Enum>
      | 			</EnumInfo>
      | 			<EnumInfo>
      | 				<Text><![CDATA[Stopping]]></Text>
      | 				<Enum>3</Enum>
      | 			</EnumInfo>
      | 			<EnumInfo>
      | 				<Text><![CDATA[StartError]]></Text>
      | 				<Enum>4</Enum>
      | 			</EnumInfo>
      | 			<EnumInfo>
      | 				<Text><![CDATA[StopError]]></Text>
      | 				<Enum>5</Enum>
      | 			</EnumInfo>
      | 			<Hides>
      | 				<Hide GUID="{BEEA3766-C152-4B4D-80E7-6332297C102B}"/>
      | 			</Hides>
      | 		</DataType>
      | 		<DataType>
      | 			<Name GUID="{BCEA2DD9-BE3C-4A28-A404-258B4399FDEA}" Namespace="TcDataExchange">ITcStreamAdsNotificationHandler</Name>
      | 			<BitSize X64="64">32</BitSize>
      | 			<BaseType GUID="{00000001-0000-0000-E000-000000000064}">ITcUnknown</BaseType>
      | 			<Method>
      | 				<Name>Start</Name>
      | 				<ReturnType GUID="{18071995-0000-0000-0000-000000000019}">HRESULT</ReturnType>
      | 				<ReturnBitSize>32</ReturnBitSize>
      | 				<Parameter>
      | 					<Name>sampleTime100ns</Name>
      | 					<Comment><![CDATA[SampleTime in 100ns. If the value is 0 or too small, the requests will be send as fast as possible.]]></Comment>
      | 					<Type GUID="{18071995-0000-0000-0000-000000000008}" Optional="0">UDINT</Type>
      | 					<BitSize>32</BitSize>
      | 				</Parameter>
      | 				<Parameter>
      | 					<Name>delayTime100ns</Name>
      | 					<Comment><![CDATA[DelayTime in 100ns.]]></Comment>
      | 					<Type GUID="{18071995-0000-0000-0000-000000000008}" Optional="10">UDINT</Type>
      | 					<BitSize>32</BitSize>
      | 				</Parameter>
      | 				<Parameter>
      | 					<Name>createTimeoutMs</Name>
      | 					<Type GUID="{18071995-0000-0000-0000-000000000006}" Optional="1000">INT</Type>
      | 					<BitSize>16</BitSize>
      | 				</Parameter>
      | 				<Parameter>
      | 					<Name>transMode</Name>
      | 					<Type GUID="{2919D6B4-47C4-4AE8-B706-E94C497ECB99}" Namespace="TcDataExchange" Optional="0">NotificationTransMode</Type>
      | 					<BitSize>16</BitSize>
      | 				</Parameter>
      | 			</Method>
      | 			<Method>
      | 				<Name>Stop</Name>
      | 				<ReturnType GUID="{18071995-0000-0000-0000-000000000019}">HRESULT</ReturnType>
      | 				<ReturnBitSize>32</ReturnBitSize>
      | 				<Parameter>
      | 					<Name>stopTimeoutMs</Name>
      | 					<Type GUID="{18071995-0000-0000-0000-000000000006}" Optional="1000">INT</Type>
      | 					<BitSize>16</BitSize>
      | 				</Parameter>
      | 			</Method>
      | 			<Method>
      | 				<Name>GetState</Name>
      | 				<ReturnType GUID="{18071995-0000-0000-0000-000000000019}">HRESULT</ReturnType>
      | 				<ReturnBitSize>32</ReturnBitSize>
      | 				<Parameter>
      | 					<Name>pState</Name>
      | 					<Type GUID="{B75DDCED-7BC8-45F5-8D80-27345642612D}" Namespace="TcDataExchange" PointerTo="1">NotificationState</Type>
      | 					<BitSize X64="64">32</BitSize>
      | 				</Parameter>
      | 				<Parameter>
      | 					<Name>pErrorCode</Name>
      | 					<Type GUID="{18071995-0000-0000-0000-000000000009}" PointerTo="1">DINT</Type>
      | 					<BitSize X64="64">32</BitSize>
      | 				</Parameter>
      | 			</Method>
      | 			<Method>
      | 				<Name>WaitFor</Name>
      | 				<ReturnType GUID="{18071995-0000-0000-0000-000000000019}">HRESULT</ReturnType>
      | 				<ReturnBitSize>32</ReturnBitSize>
      | 				<Parameter>
      | 					<Name>targetState</Name>
      | 					<Type GUID="{B75DDCED-7BC8-45F5-8D80-27345642612D}" Namespace="TcDataExchange">NotificationState</Type>
      | 					<BitSize>16</BitSize>
      | 				</Parameter>
      | 				<Parameter>
      | 					<Name>wait</Name>
      | 					<Type GUID="{18071995-0000-0000-0000-000000000030}" Optional="1">BOOL</Type>
      | 					<BitSize>8</BitSize>
      | 				</Parameter>
      | 			</Method>
      | 			<Method>
      | 				<Name>LastIndicationTime</Name>
      | 				<ReturnType GUID="{18071995-0000-0000-0000-000000000019}">HRESULT</ReturnType>
      | 				<ReturnBitSize>32</ReturnBitSize>
      | 				<Parameter>
      | 					<Name>pTimestamp</Name>
      | 					<Type GUID="{18071995-0000-0000-0000-00000000000C}" PointerTo="1">LINT</Type>
      | 					<BitSize X64="64">32</BitSize>
      | 				</Parameter>
      | 			</Method>
      | 			<Hides>
      | 				<Hide GUID="{0FD54C3A-649C-4819-BA34-40090DB2854F}"/>
      | 				<Hide GUID="{B851627D-4078-4428-873B-9E0DE756697F}"/>
      | 				<Hide GUID="{82738EA0-63AE-4386-9AC8-D5A166BE7CE6}"/>
      | 				<Hide GUID="{62C58600-337E-4913-B519-B241B47A093F}"/>
      | 				<Hide GUID="{F19E62E1-3672-44A5-AE6F-41D70903D13E}"/>
      | 				<Hide GUID="{188DFF90-A46E-4A6C-BF2A-4B79F1A4A7D7}"/>
      | 				<Hide GUID="{20D7666F-EA21-4A02-B0BF-92A2B39D0282}"/>
      | 				<Hide GUID="{B6680295-EE8B-49D4-B982-46287CB9DC7F}"/>
      | 				<Hide GUID="{640F79DB-CF38-45B7-A5A6-1F8ACF6E88C7}"/>
      | 				<Hide GUID="{ACD4E2BC-BCCF-47C3-994A-79C84DA897B4}"/>
      | 				<Hide GUID="{CA600548-350B-4000-92EC-05CC4A5FC0D9}"/>
      | 			</Hides>
      | 		</DataType>
      | 		<DataType>
      | 			<Name GUID="{E2F9B58E-D9A1-47B2-8E7C-99E63D58AA89}" Namespace="TcDataExchange">ITcStreamAdsClient</Name>
      | 			<BitSize X64="64">32</BitSize>
      | 			<BaseType GUID="{00000001-0000-0000-E000-000000000064}">ITcUnknown</BaseType>
      | 			<Method>
      | 				<Name>CreateReadRequest</Name>
      | 				<ReturnType GUID="{18071995-0000-0000-0000-000000000019}">HRESULT</ReturnType>
      | 				<ReturnBitSize>32</ReturnBitSize>
      | 				<Parameter>
      | 					<Name>parentOid</Name>
      | 					<Type GUID="{18071995-0000-0000-0000-00000000000F}">OTCID</Type>
      | 					<BitSize>32</BitSize>
      | 				</Parameter>
      | 				<Parameter>
      | 					<Name>ppRequestHandler</Name>
      | 					<Type GUID="{3BC82419-4CB4-48F5-8384-E3D86DEA2DAE}" Namespace="TcDataExchange" PointerTo="1" RpcDirection="out">ITcStreamAdsRequestHandler</Type>
      | 					<BitSize X64="64">32</BitSize>
      | 				</Parameter>
      | 				<Parameter>
      | 					<Name>amsAddr</Name>
      | 					<Type GUID="{18071995-0000-0000-0000-000000000042}" RpcDirection="in">AMSADDR</Type>
      | 					<BitSize>64</BitSize>
      | 				</Parameter>
      | 				<Parameter>
      | 					<Name>idxGrp</Name>
      | 					<Type GUID="{18071995-0000-0000-0000-000000000008}" RpcDirection="in">UDINT</Type>
      | 					<BitSize>32</BitSize>
      | 				</Parameter>
      | 				<Parameter>
      | 					<Name>idxOffs</Name>
      | 					<Type GUID="{18071995-0000-0000-0000-000000000008}" RpcDirection="in">UDINT</Type>
      | 					<BitSize>32</BitSize>
      | 				</Parameter>
      | 				<Parameter>
      | 					<Name>byteSize</Name>
      | 					<Type GUID="{18071995-0000-0000-0000-000000000008}" RpcDirection="in">UDINT</Type>
      | 					<BitSize>32</BitSize>
      | 				</Parameter>
      | 				<Parameter>
      | 					<Name>pSink</Name>
      | 					<Type GUID="{CD026BE9-DD1E-4238-B09F-CDE426934EFB}" Namespace="TcDataExchange" RpcDirection="in">ITcStreamSyncDataSink</Type>
      | 					<BitSize X64="64">32</BitSize>
      | 				</Parameter>
      | 			</Method>
      | 			<Method>
      | 				<Name>CreateWriteRequest</Name>
      | 				<ReturnType GUID="{18071995-0000-0000-0000-000000000019}">HRESULT</ReturnType>
      | 				<ReturnBitSize>32</ReturnBitSize>
      | 				<Parameter>
      | 					<Name>parentOid</Name>
      | 					<Type GUID="{18071995-0000-0000-0000-00000000000F}">OTCID</Type>
      | 					<BitSize>32</BitSize>
      | 				</Parameter>
      | 				<Parameter>
      | 					<Name>ppRequestHandler</Name>
      | 					<Type GUID="{3BC82419-4CB4-48F5-8384-E3D86DEA2DAE}" Namespace="TcDataExchange" PointerTo="1" RpcDirection="out">ITcStreamAdsRequestHandler</Type>
      | 					<BitSize X64="64">32</BitSize>
      | 				</Parameter>
      | 				<Parameter>
      | 					<Name>amsAddr</Name>
      | 					<Type GUID="{18071995-0000-0000-0000-000000000042}" RpcDirection="in">AMSADDR</Type>
      | 					<BitSize>64</BitSize>
      | 				</Parameter>
      | 				<Parameter>
      | 					<Name>idxGrp</Name>
      | 					<Type GUID="{18071995-0000-0000-0000-000000000008}" RpcDirection="in">UDINT</Type>
      | 					<BitSize>32</BitSize>
      | 				</Parameter>
      | 				<Parameter>
      | 					<Name>idxOffs</Name>
      | 					<Type GUID="{18071995-0000-0000-0000-000000000008}" RpcDirection="in">UDINT</Type>
      | 					<BitSize>32</BitSize>
      | 				</Parameter>
      | 				<Parameter>
      | 					<Name>byteSize</Name>
      | 					<Type GUID="{18071995-0000-0000-0000-000000000008}" RpcDirection="in">UDINT</Type>
      | 					<BitSize>32</BitSize>
      | 				</Parameter>
      | 				<Parameter>
      | 					<Name>pSource</Name>
      | 					<Type GUID="{877CB26F-4EC1-469B-9F87-706DDBDA821F}" Namespace="TcDataExchange" RpcDirection="in">ITcStreamSyncDataSource</Type>
      | 					<BitSize X64="64">32</BitSize>
      | 				</Parameter>
      | 			</Method>
      | 			<Method>
      | 				<Name>CreateReadWriteRequest</Name>
      | 				<ReturnType GUID="{18071995-0000-0000-0000-000000000019}">HRESULT</ReturnType>
      | 				<ReturnBitSize>32</ReturnBitSize>
      | 				<Parameter>
      | 					<Name>parentOid</Name>
      | 					<Type GUID="{18071995-0000-0000-0000-00000000000F}">OTCID</Type>
      | 					<BitSize>32</BitSize>
      | 				</Parameter>
      | 				<Parameter>
      | 					<Name>ppRequestHandler</Name>
      | 					<Type GUID="{3BC82419-4CB4-48F5-8384-E3D86DEA2DAE}" Namespace="TcDataExchange" PointerTo="1" RpcDirection="out">ITcStreamAdsRequestHandler</Type>
      | 					<BitSize X64="64">32</BitSize>
      | 				</Parameter>
      | 				<Parameter>
      | 					<Name>amsAddr</Name>
      | 					<Type GUID="{18071995-0000-0000-0000-000000000042}" RpcDirection="in">AMSADDR</Type>
      | 					<BitSize>64</BitSize>
      | 				</Parameter>
      | 				<Parameter>
      | 					<Name>idxGrp</Name>
      | 					<Type GUID="{18071995-0000-0000-0000-000000000008}" RpcDirection="in">UDINT</Type>
      | 					<BitSize>32</BitSize>
      | 				</Parameter>
      | 				<Parameter>
      | 					<Name>idxOffs</Name>
      | 					<Type GUID="{18071995-0000-0000-0000-000000000008}" RpcDirection="in">UDINT</Type>
      | 					<BitSize>32</BitSize>
      | 				</Parameter>
      | 				<Parameter>
      | 					<Name>writeSize</Name>
      | 					<Type GUID="{18071995-0000-0000-0000-000000000008}" RpcDirection="in">UDINT</Type>
      | 					<BitSize>32</BitSize>
      | 				</Parameter>
      | 				<Parameter>
      | 					<Name>pSource</Name>
      | 					<Type GUID="{877CB26F-4EC1-469B-9F87-706DDBDA821F}" Namespace="TcDataExchange" RpcDirection="in">ITcStreamSyncDataSource</Type>
      | 					<BitSize X64="64">32</BitSize>
      | 				</Parameter>
      | 				<Parameter>
      | 					<Name>readSize</Name>
      | 					<Type GUID="{18071995-0000-0000-0000-000000000008}" RpcDirection="in">UDINT</Type>
      | 					<BitSize>32</BitSize>
      | 				</Parameter>
      | 				<Parameter>
      | 					<Name>pSink</Name>
      | 					<Type GUID="{CD026BE9-DD1E-4238-B09F-CDE426934EFB}" Namespace="TcDataExchange" RpcDirection="in">ITcStreamSyncDataSink</Type>
      | 					<BitSize X64="64">32</BitSize>
      | 				</Parameter>
      | 			</Method>
      | 			<Method>
      | 				<Name>CreateNotificationHandler</Name>
      | 				<ReturnType GUID="{18071995-0000-0000-0000-000000000019}">HRESULT</ReturnType>
      | 				<ReturnBitSize>32</ReturnBitSize>
      | 				<Parameter>
      | 					<Name>parentOid</Name>
      | 					<Type GUID="{18071995-0000-0000-0000-00000000000F}">OTCID</Type>
      | 					<BitSize>32</BitSize>
      | 				</Parameter>
      | 				<Parameter>
      | 					<Name>ppNotificationHandler</Name>
      | 					<Type GUID="{BCEA2DD9-BE3C-4A28-A404-258B4399FDEA}" Namespace="TcDataExchange" PointerTo="1" RpcDirection="out">ITcStreamAdsNotificationHandler</Type>
      | 					<BitSize X64="64">32</BitSize>
      | 				</Parameter>
      | 				<Parameter>
      | 					<Name>amsAddr</Name>
      | 					<Type GUID="{18071995-0000-0000-0000-000000000042}">AMSADDR</Type>
      | 					<BitSize>64</BitSize>
      | 				</Parameter>
      | 				<Parameter>
      | 					<Name>idxGrp</Name>
      | 					<Type GUID="{18071995-0000-0000-0000-000000000008}" RpcDirection="in">UDINT</Type>
      | 					<BitSize>32</BitSize>
      | 				</Parameter>
      | 				<Parameter>
      | 					<Name>idxOffs</Name>
      | 					<Type GUID="{18071995-0000-0000-0000-000000000008}" RpcDirection="in">UDINT</Type>
      | 					<BitSize>32</BitSize>
      | 				</Parameter>
      | 				<Parameter>
      | 					<Name>byteSize</Name>
      | 					<Type GUID="{18071995-0000-0000-0000-000000000008}" RpcDirection="in">UDINT</Type>
      | 					<BitSize>32</BitSize>
      | 				</Parameter>
      | 				<Parameter>
      | 					<Name>pSink</Name>
      | 					<Type GUID="{CD026BE9-DD1E-4238-B09F-CDE426934EFB}" Namespace="TcDataExchange" RpcDirection="in">ITcStreamSyncDataSink</Type>
      | 					<BitSize X64="64">32</BitSize>
      | 				</Parameter>
      | 			</Method>
      | 			<Method>
      | 				<Name>CheckOrders</Name>
      | 				<ReturnType GUID="{18071995-0000-0000-0000-000000000019}">HRESULT</ReturnType>
      | 				<ReturnBitSize>32</ReturnBitSize>
      | 			</Method>
      | 			<Hides>
      | 				<Hide GUID="{E5572F78-39F4-4573-890C-3DF0E2006105}"/>
      | 				<Hide GUID="{52252529-8C17-45D1-85B4-6A458C0F3E94}"/>
      | 				<Hide GUID="{F824C7E1-F0C6-44A6-B482-897B83EFF54D}"/>
      | 				<Hide GUID="{89D1DEF9-1EDB-4DC7-B44F-67745448E326}"/>
      | 				<Hide GUID="{9AF2891A-A1C3-41B4-843B-F1318836B90C}"/>
      | 				<Hide GUID="{C92F8EE8-70FC-4938-AE5D-0804054FE778}"/>
      | 				<Hide GUID="{692D2F91-2921-429B-A2FD-B23E2D06FE57}"/>
      | 				<Hide GUID="{247F4AE9-8FC4-4311-BF3B-2963D4FB048A}"/>
      | 				<Hide GUID="{FB8AA9BF-37B4-4992-B5AC-BBA0F4D43373}"/>
      | 				<Hide GUID="{7427C36F-E349-41A6-A066-CB0C042DD556}"/>
      | 				<Hide GUID="{E46C7F48-0073-45AF-850A-7F1CB9D0F1BC}"/>
      | 				<Hide GUID="{096DB961-B576-4662-AA01-00D308385BF0}"/>
      | 				<Hide GUID="{A0AD0C9E-66BD-49F7-B782-910B430A1CD8}"/>
      | 				<Hide GUID="{FA6AC3AF-43AA-44CB-BA36-5723B1AD464D}"/>
      | 				<Hide GUID="{0614F527-21B4-4192-AE03-7FDCC97AD564}"/>
      | 				<Hide GUID="{20F9385A-0313-4208-B227-DA4EACC1424F}"/>
      | 				<Hide GUID="{DBEA0444-99ED-4B99-9B51-31DB70AF46EF}"/>
      | 				<Hide GUID="{C3B2FC5E-7AD1-45D8-9723-AA6C61AD9B60}"/>
      | 				<Hide GUID="{CF97D717-7515-4E5A-BE1F-84F5A676B8F8}"/>
      | 				<Hide GUID="{B3BDED57-1312-4D96-B06F-2628ECBA6EEF}"/>
      | 				<Hide GUID="{5DE91436-84B1-4D76-B0CA-1D6620CA428C}"/>
      | 				<Hide GUID="{A0E457C6-B984-4427-829D-FA992FA6D9F8}"/>
      | 				<Hide GUID="{49669A99-FF7E-4056-9658-FDC96AB6BD99}"/>
      | 				<Hide GUID="{53867E37-5FD2-456B-BE41-4F337E21E47A}"/>
      | 				<Hide GUID="{A3973658-0AF9-4706-9520-0AAF0F575BFE}"/>
      | 				<Hide GUID="{FC062AA8-EE46-46C7-94CF-827603675385}"/>
      | 				<Hide GUID="{021F7DA4-A9B9-4EF5-80F9-A8DBC397B675}"/>
      | 				<Hide GUID="{4D5006B6-E8E6-4498-9498-ACA7E948FC8F}"/>
      | 				<Hide GUID="{984AB404-08AC-4281-AB66-6ED5B3F17DFE}"/>
      | 				<Hide GUID="{D581F6CF-93AC-4E4B-8D6F-3F0EF3492A71}"/>
      | 				<Hide GUID="{7A32D7B0-99BA-4055-815F-11160248ACD0}"/>
      | 				<Hide GUID="{9E7FC559-CAD5-43C8-B16B-2E56C1991573}"/>
      | 				<Hide GUID="{F062CF59-8FAE-4FCB-A01C-9B649900BCA5}"/>
      | 				<Hide GUID="{8728E0D9-0A46-4A30-9F10-DD1BF2EA33CE}"/>
      | 				<Hide GUID="{DFBB006E-343D-4910-A9C8-3AB2FE1535D3}"/>
      | 				<Hide GUID="{28C016BE-C467-4209-83F6-DED24711BF6D}"/>
      | 				<Hide GUID="{090DBC60-C9BC-4AB3-B82F-77F59E060169}"/>
      | 				<Hide GUID="{7C69CB05-063E-4BC5-9379-7224930A2D33}"/>
      | 				<Hide GUID="{AFAD7A5B-01FD-4391-87A6-15283DC78C95}"/>
      | 				<Hide GUID="{5E61A921-550A-4063-9429-A8A28DE5A1E3}"/>
      | 				<Hide GUID="{6BB012C3-FEAE-471E-BD95-27EDA5BB3A24}"/>
      | 				<Hide GUID="{E5B9394C-8543-4D1E-86CA-EC772D80F874}"/>
      | 				<Hide GUID="{B8FC3674-8C27-4962-8D53-5010B3276572}"/>
      | 				<Hide GUID="{7A879166-081C-4396-83F5-1ED6DDC3FE02}"/>
      | 				<Hide GUID="{906345FE-D08D-48EB-B8DC-3909739597CB}"/>
      | 				<Hide GUID="{D3B5497D-2C29-4E09-AE6E-7107BDE26921}"/>
      | 				<Hide GUID="{584A9F4B-B4B2-498C-8C91-9E721AEE609C}"/>
      | 			</Hides>
      | 		</DataType>
      | 		<DataType>
      | 			<Name GUID="{D43C781F-D2A3-47F2-828C-7AB11F3EB7CF}" Namespace="TcDataExchange">ITcStreamSymbolInterfaceConnector</Name>
      | 			<BitSize X64="64">32</BitSize>
      | 			<BaseType GUID="{00000001-0000-0000-E000-000000000064}">ITcUnknown</BaseType>
      | 			<Method>
      | 				<Name>WriteData</Name>
      | 				<ReturnType GUID="{18071995-0000-0000-0000-000000000019}">HRESULT</ReturnType>
      | 				<ReturnBitSize>32</ReturnBitSize>
      | 				<Parameter>
      | 					<Name>portId</Name>
      | 					<Type GUID="{18071995-0000-0000-0000-000000000008}" RpcDirection="in">UDINT</Type>
      | 					<BitSize>32</BitSize>
      | 				</Parameter>
      | 				<Parameter>
      | 					<Name>size</Name>
      | 					<Type GUID="{18071995-0000-0000-0000-000000000008}" RpcDirection="in">UDINT</Type>
      | 					<BitSize>32</BitSize>
      | 				</Parameter>
      | 				<Parameter>
      | 					<Name>data</Name>
      | 					<Type GUID="{18071995-0000-0000-0000-000000000001}" PointerTo="1" RpcDirection="in">BYTE</Type>
      | 					<BitSize X64="64">32</BitSize>
      | 				</Parameter>
      | 			</Method>
      | 			<Method>
      | 				<Name>ReadData</Name>
      | 				<ReturnType GUID="{18071995-0000-0000-0000-000000000019}">HRESULT</ReturnType>
      | 				<ReturnBitSize>32</ReturnBitSize>
      | 				<Parameter>
      | 					<Name>portId</Name>
      | 					<Type GUID="{18071995-0000-0000-0000-000000000008}" RpcDirection="in">UDINT</Type>
      | 					<BitSize>32</BitSize>
      | 				</Parameter>
      | 				<Parameter>
      | 					<Name>size</Name>
      | 					<Type GUID="{18071995-0000-0000-0000-000000000008}" RpcDirection="in">UDINT</Type>
      | 					<BitSize>32</BitSize>
      | 				</Parameter>
      | 				<Parameter>
      | 					<Name>data</Name>
      | 					<Type GUID="{18071995-0000-0000-0000-000000000001}" PointerTo="1" RpcDirection="out">BYTE</Type>
      | 					<BitSize X64="64">32</BitSize>
      | 				</Parameter>
      | 			</Method>
      | 		</DataType>
      | 		<DataType>
      | 			<Name GUID="{F19BC36D-E8D2-4B1C-8F2C-B31A287B0759}" HideSubItems="true">OutputsArray</Name>
      | 			<BitSize>7392</BitSize>
      | 			<BaseType GUID="{18071995-0000-0000-0000-000000000001}">BYTE</BaseType>
      | 			<ArrayInfo>
      | 				<LBound>0</LBound>
      | 				<Elements>924</Elements>
      | 			</ArrayInfo>
      | 		</DataType>
      | 	</DataTypes>
      | 	<Translations/>
      | 	<System>
      | 		<Tasks>
      | 			<Task ObjectId="33620000" CycleTime="100000" AmsPort="350" Priority="20">
      | 				<Name>TcDataExchangeModulesTask</Name>
      | 			</Task>
      | 		</Tasks>
      | 		<Modules>
      | 			<Module GUID="{E38BFC78-135A-4B90-A7E9-B3ECAB89AD55}" ClassFactoryId="Beckhoff Automation GmbH|TcDataExchangeModules|1.1.24.0" Group="DataExchange|Protocols">
      | 				<Name>AdsClient</Name>
      | 				<CLSID ClassFactory="TcDataExchangeModules" RealTimeInstantiable="true">{E38BFC78-135A-4B90-A7E9-B3ECAB89AD55}</CLSID>
      | 				<Info/>
      | 				<InitSequence>PSO</InitSequence>
      | 				<Contexts>
      | 					<Context>
      | 						<Id>1</Id>
      | 					</Context>
      | 				</Contexts>
      | 				<Interfaces>
      | 					<Interface DisableCodeGeneration="true">
      | 						<Type GUID="{00000012-0000-0000-E000-000000000064}">ITComObject</Type>
      | 					</Interface>
      | 					<Interface DisableCodeGeneration="true">
      | 						<Type GUID="{03000012-0000-0000-E000-000000000064}">ITcADI</Type>
      | 					</Interface>
      | 					<Interface DisableCodeGeneration="true">
      | 						<Type GUID="{03000018-0000-0000-E000-000000000064}">ITcWatchSource</Type>
      | 					</Interface>
      | 					<Interface>
      | 						<Type GUID="{E2F9B58E-D9A1-47B2-8E7C-99E63D58AA89}" Namespace="TcDataExchange">ITcStreamAdsClient</Type>
      | 					</Interface>
      | 				</Interfaces>
      | 				<Parameters>
      | 					<Parameter OnlineParameter="true" DisableCodeGeneration="true" ReadOnly="true">
      | 						<Name>LocalNetId</Name>
      | 						<BitSize>48</BitSize>
      | 						<BaseType GUID="{18071995-0000-0000-0000-000000000041}">AMSNETID</BaseType>
      | 						<PTCID>#x00000001</PTCID>
      | 						<ContextId>1</ContextId>
      | 					</Parameter>
      | 					<Parameter>
      | 						<Name>LocalPortNo</Name>
      | 						<BitSize>16</BitSize>
      | 						<BaseType GUID="{18071995-0000-0000-0000-000000000005}">UINT</BaseType>
      | 						<Default>
      | 							<Value>0</Value>
      | 						</Default>
      | 						<PTCID>#x00000002</PTCID>
      | 						<ContextId>1</ContextId>
      | 					</Parameter>
      | 					<Parameter>
      | 						<Name>LocalPortName</Name>
      | 						<BitSize>256</BitSize>
      | 						<BaseType GUID="{18071995-0000-0000-0000-00010000001F}">STRING(31)</BaseType>
      | 						<PTCID>#x00000003</PTCID>
      | 						<ContextId>1</ContextId>
      | 					</Parameter>
      | 					<Parameter HideParameter="true">
      | 						<Name>TraceLevelMax</Name>
      | 						<Comment TxtId=""><![CDATA[Controls the amount of log messages.]]></Comment>
      | 						<BitSize>32</BitSize>
      | 						<BaseType GUID="{8007AE3B-86BB-40F2-B385-EF87FCC239A4}">TcTraceLevel</BaseType>
      | 						<PTCID>#x03002103</PTCID>
      | 						<ContextId>1</ContextId>
      | 					</Parameter>
      | 					<Parameter HideParameter="true">
      | 						<Name>Proxy</Name>
      | 						<BitSize>64</BitSize>
      | 						<BaseType GUID="{18071995-0000-0000-0000-00000000000B}">ULINT</BaseType>
      | 						<PTCID>#x000000f1</PTCID>
      | 					</Parameter>
      | 				</Parameters>
      | 				<InstanceName>AdsClient</InstanceName>
      | 				<OTCID>#x01010010</OTCID>
      | 				<ParameterValues>
      | 					<Value>
      | 						<Name>LocalPortNo</Name>
      | 						<Value>0</Value>
      | 					</Value>
      | 					<Value>
      | 						<Name>LocalPortName</Name>
      | 						<String/>
      | 					</Value>
      | 					<Value>
      | 						<Name>TraceLevelMax</Name>
      | 						<EnumText>tlAlways</EnumText>
      | 					</Value>
      | 					<Value>
      | 						<Name>Proxy</Name>
      | 						<Value>0</Value>
      | 					</Value>
      | 				</ParameterValues>
      | 			</Module>
      | 			<Module GUID="{4D013B77-597F-47DA-A44F-925F710443F1}" ClassFactoryId="Beckhoff Automation GmbH|TcDataExchangeModules|1.1.24.0" Group="DataExchange|Protocols">
      | 				<Name>SymbolInterfaceConnector</Name>
      | 				<CLSID ClassFactory="TcDataExchangeModules">{4D013B77-597F-47DA-A44F-925F710443F1}</CLSID>
      | 				<Info/>
      | 				<InitSequence>PSO</InitSequence>
      | 				<Contexts>
      | 					<Context>
      | 						<Id>1</Id>
      | 					</Context>
      | 				</Contexts>
      | 				<Interfaces>
      | 					<Interface DisableCodeGeneration="true">
      | 						<Type GUID="{00000012-0000-0000-E000-000000000064}">ITComObject</Type>
      | 					</Interface>
      | 					<Interface DisableCodeGeneration="true">
      | 						<Type GUID="{03000012-0000-0000-E000-000000000064}">ITcADI</Type>
      | 					</Interface>
      | 					<Interface DisableCodeGeneration="true">
      | 						<Type GUID="{03000018-0000-0000-E000-000000000064}">ITcWatchSource</Type>
      | 					</Interface>
      | 					<Interface>
      | 						<Type GUID="{D43C781F-D2A3-47F2-828C-7AB11F3EB7CF}" Namespace="TcDataExchange">ITcStreamSymbolInterfaceConnector</Type>
      | 					</Interface>
      | 				</Interfaces>
      | 				<Parameters>
      | 					<Parameter HideParameter="true">
      | 						<Name>TraceLevelMax</Name>
      | 						<Comment TxtId=""><![CDATA[Controls the amount of log messages.]]></Comment>
      | 						<BitSize>32</BitSize>
      | 						<BaseType GUID="{8007AE3B-86BB-40F2-B385-EF87FCC239A4}">TcTraceLevel</BaseType>
      | 						<PTCID>#x03002103</PTCID>
      | 						<ContextId>1</ContextId>
      | 					</Parameter>
      | 					<Parameter>
      | 						<Name>InputSyncBuffers</Name>
      | 						<BitSize>0</BitSize>
      | 						<BaseType GUID="{18071995-0000-0000-0000-00000000000F}">OTCID</BaseType>
      | 						<ArrayInfo>
      | 							<LBound>0</LBound>
      | 							<Elements Min="0" MaxUnbounded="true">0</Elements>
      | 						</ArrayInfo>
      | 						<PTCID>#x00000001</PTCID>
      | 						<ContextId>1</ContextId>
      | 					</Parameter>
      | 					<Parameter>
      | 						<Name>OutputSyncBuffers</Name>
      | 						<BitSize>0</BitSize>
      | 						<BaseType GUID="{18071995-0000-0000-0000-00000000000F}">OTCID</BaseType>
      | 						<ArrayInfo>
      | 							<LBound>0</LBound>
      | 							<Elements Min="0" MaxUnbounded="true">0</Elements>
      | 						</ArrayInfo>
      | 						<PTCID>#x00000002</PTCID>
      | 						<ContextId>1</ContextId>
      | 					</Parameter>
      | 					<Parameter HideParameter="true">
      | 						<Name>Outputs</Name>
      | 						<BitSize>7392</BitSize>
      | 						<BaseType GUID="{F19BC36D-E8D2-4B1C-8F2C-B31A287B0759}">OutputsArray</BaseType>
      | 						<ArrayInfo>
      | 							<LBound>0</LBound>
      | 							<Elements>1</Elements>
      | 						</ArrayInfo>
      | 						<PTCID>#x000000f6</PTCID>
      | 					</Parameter>
      | 				</Parameters>
      | 				<InterfacePointers>
      | 					<InterfacePointer>
      | 						<PTCID>#x00000003</PTCID>
      | 						<Name>Synchronizer</Name>
      | 						<Type GUID="{9165C8A1-78D1-4B81-89D0-BA48F61AF93B}" Namespace="TcDataExchange">ITcStreamSynchronizer</Type>
      | 						<ContextId>1</ContextId>
      | 					</InterfacePointer>
      | 					<InterfacePointer>
      | 						<PTCID>#x00000004</PTCID>
      | 						<Name>AdsClient</Name>
      | 						<Type GUID="{E2F9B58E-D9A1-47B2-8E7C-99E63D58AA89}" Namespace="TcDataExchange">ITcStreamAdsClient</Type>
      | 						<ContextId>1</ContextId>
      | 					</InterfacePointer>
      | 					<InterfacePointer>
      | 						<PTCID>#x03002060</PTCID>
      | 						<Name>CyclicCaller</Name>
      | 						<Type GUID="{0300001E-0000-0000-E000-000000000064}">ITcCyclicCaller</Type>
      | 						<ContextId>1</ContextId>
      | 					</InterfacePointer>
      | 				</InterfacePointers>
      | 				<InstanceName>SymbolInterfaceConnector</InstanceName>
      | 				<OTCID>#x01010020</OTCID>
      | 				<ParameterValues>
      | 					<Value>
      | 						<Name>TraceLevelMax</Name>
      | 						<EnumText>tlAlways</EnumText>
      | 					</Value>
      | 					<Value>
      | 						<Name>Outputs[0]</Name>
      | 						<Data>000000000400000032000000a086010003000000060000008027c8a40101530300000000000000004d41494e2e666243617274657369616e4a6f79737469632e66584178697300000000000000000000000000000000000000000000000000000000000000000000000000000000000000000000000000000000000000000000000000000000000000000000000000000000000000000000000000000000000000000000000000000000000000000000000000000000000000000000000000000000000000000000000000000000000000000000000000000000000000000000000000000000000000000000000000000000000000000000000000000000000000000000000000000000000000000000000000000000000000000000000000000000000000000000e80300000100030040420f00010000000400000032000000a086010003000000060000008027c8a40101530300000000000000004d41494e2e666243617274657369616e4a6f79737469632e66594178697300000000000000000000000000000000000000000000000000000000000000000000000000000000000000000000000000000000000000000000000000000000000000000000000000000000000000000000000000000000000000000000000000000000000000000000000000000000000000000000000000000000000000000000000000000000000000000000000000000000000000000000000000000000000000000000000000000000000000000000000000000000000000000000000000000000000000000000000000000000000000000000000000000000000000000000e80300000100030040420f00020000000400000032000000a086010003000000060000008027c8a40101530300000000000000004d41494e2e666243617274657369616e4a6f79737469632e665a4178697300000000000000000000000000000000000000000000000000000000000000000000000000000000000000000000000000000000000000000000000000000000000000000000000000000000000000000000000000000000000000000000000000000000000000000000000000000000000000000000000000000000000000000000000000000000000000000000000000000000000000000000000000000000000000000000000000000000000000000000000000000000000000000000000000000000000000000000000000000000000000000000000000000000000000000000e80300000100030040420f00</Data>
      | 					</Value>
      | 				</ParameterValues>
      | 				<InterfacePointerValues>
      | 					<Value>
      | 						<Name>Synchronizer</Name>
      | 						<OTCID>#x00000000</OTCID>
      | 					</Value>
      | 					<Value>
      | 						<Name>AdsClient</Name>
      | 						<OTCID>#x01010010</OTCID>
      | 					</Value>
      | 					<Value>
      | 						<Name>CyclicCaller</Name>
      | 						<OTCID>#x02010020</OTCID>
      | 					</Value>
      | 				</InterfacePointerValues>
      | 			</Module>
      | 		</Modules>
      | 	</System>
      | </TcRuntimAdapterProject>
      SymbolInterfaceInfo=|
      | <PortInfo>
      | 	<Inputs>
      | 		<SymbolControlItems/>
      | 	</Inputs>
      | 	<Outputs>
      | 		<SymbolControlItems>
      | 			<SymbolControlItem GroupName="ADS Read" GroupDescription="Parameters for ADS Read command">
      | 				<Parameters>
      | 					<Parameter Name="Name">MAIN.fbCartesianJoystic.fXAxis</Parameter>
      | 					<Parameter Name="SymbolName">MAIN.fbCartesianJoystic.fXAxis</Parameter>
      | 					<Parameter Name="SymbolType">REAL</Parameter>
      | 					<Parameter Name="SymbolGuid">{18071995-0000-0000-0000-00000000000D}</Parameter>
      | 					<Parameter Name="AmsNetId">128.39.200.164.1.1</Parameter>
      | 					<Parameter Name="Port">851</Parameter>
      | 					<Parameter Name="IndexGroup">#x0</Parameter>
      | 					<Parameter Name="IndexOffset">#x0</Parameter>
      | 					<Parameter Name="BitSize">32</Parameter>
      | 					<Parameter Name="InterpolationMode">3</Parameter>
      | 					<Parameter Name="ExtrapolationMode">0</Parameter>
      | 					<Parameter Name="SymbolInfo">0300400000000000000000000100000078000000D0070000E9FD00001600000000000000000000000000000000000000000000000000000000000000000000007800000001000000000000000000000004000000000000000400000081100000040000000000000000005245414C0000009519071800000000000000000000000D02000F06446973706C61794D696E56616C7565002D3130303030000F05446973706C61794D617856616C75650031303030300000000000</Parameter>
      | 					<Parameter Name="TargetPlatform">1</Parameter>
      | 					<Parameter Name="SampleTime TC[100ns]">100000</Parameter>
      | 					<Parameter Name="SampleTime">100000</Parameter>
      | 					<Parameter Name="ReadViaNotification">True</Parameter>
      | 					<Parameter Name="Transmode">3</Parameter>
      | 					<Parameter Name="Timeout">1000</Parameter>
      | 					<Parameter Name="DelayTime">1000000</Parameter>
      | 					<Parameter Name="BufferSize">50</Parameter>
      | 					<Parameter Name="ByteSize">4</Parameter>
      | 					<Parameter Name="CodePage">65001</Parameter>
      | 				</Parameters>
      | 			</SymbolControlItem>
      | 			<SymbolControlItem GroupName="ADS Read" GroupDescription="Parameters for ADS Read command">
      | 				<Parameters>
      | 					<Parameter Name="Name">MAIN.fbCartesianJoystic.fYAxis</Parameter>
      | 					<Parameter Name="SymbolName">MAIN.fbCartesianJoystic.fYAxis</Parameter>
      | 					<Parameter Name="SymbolType">REAL</Parameter>
      | 					<Parameter Name="SymbolGuid">{18071995-0000-0000-0000-00000000000D}</Parameter>
      | 					<Parameter Name="AmsNetId">128.39.200.164.1.1</Parameter>
      | 					<Parameter Name="Port">851</Parameter>
      | 					<Parameter Name="IndexGroup">#x0</Parameter>
      | 					<Parameter Name="IndexOffset">#x0</Parameter>
      | 					<Parameter Name="BitSize">32</Parameter>
      | 					<Parameter Name="InterpolationMode">3</Parameter>
      | 					<Parameter Name="ExtrapolationMode">0</Parameter>
      | 					<Parameter Name="SymbolInfo">0300400000000000000000000100000078000000D0070000E9FD00001600000000000000000000000000000000000000000000000000000000000000000000007800000001000000000000000000000004000000000000000400000081100000040000000000000000005245414C0000009519071800000000000000000000000D02000F06446973706C61794D696E56616C7565002D3130303030000F05446973706C61794D617856616C75650031303030300000000000</Parameter>
      | 					<Parameter Name="TargetPlatform">1</Parameter>
      | 					<Parameter Name="SampleTime TC[100ns]">100000</Parameter>
      | 					<Parameter Name="SampleTime">100000</Parameter>
      | 					<Parameter Name="ReadViaNotification">True</Parameter>
      | 					<Parameter Name="Transmode">3</Parameter>
      | 					<Parameter Name="Timeout">1000</Parameter>
      | 					<Parameter Name="DelayTime">1000000</Parameter>
      | 					<Parameter Name="BufferSize">50</Parameter>
      | 					<Parameter Name="ByteSize">4</Parameter>
      | 					<Parameter Name="CodePage">65001</Parameter>
      | 				</Parameters>
      | 			</SymbolControlItem>
      | 			<SymbolControlItem GroupName="ADS Read" GroupDescription="Parameters for ADS Read command">
      | 				<Parameters>
      | 					<Parameter Name="Name">MAIN.fbCartesianJoystic.fZAxis</Parameter>
      | 					<Parameter Name="SymbolName">MAIN.fbCartesianJoystic.fZAxis</Parameter>
      | 					<Parameter Name="SymbolType">REAL</Parameter>
      | 					<Parameter Name="SymbolGuid">{18071995-0000-0000-0000-00000000000D}</Parameter>
      | 					<Parameter Name="AmsNetId">128.39.200.164.1.1</Parameter>
      | 					<Parameter Name="Port">851</Parameter>
      | 					<Parameter Name="IndexGroup">#x0</Parameter>
      | 					<Parameter Name="IndexOffset">#x0</Parameter>
      | 					<Parameter Name="BitSize">32</Parameter>
      | 					<Parameter Name="InterpolationMode">3</Parameter>
      | 					<Parameter Name="ExtrapolationMode">0</Parameter>
      | 					<Parameter Name="SymbolInfo">0300400000000000000000000100000078000000D0070000E9FD00001600000000000000000000000000000000000000000000000000000000000000000000007800000001000000000000000000000004000000000000000400000081100000040000000000000000005245414C0000009519071800000000000000000000000D02000F06446973706C61794D696E56616C7565002D3130303030000F05446973706C61794D617856616C75650031303030300000000000</Parameter>
      | 					<Parameter Name="TargetPlatform">1</Parameter>
      | 					<Parameter Name="SampleTime TC[100ns]">100000</Parameter>
      | 					<Parameter Name="SampleTime">100000</Parameter>
      | 					<Parameter Name="ReadViaNotification">True</Parameter>
      | 					<Parameter Name="Transmode">3</Parameter>
      | 					<Parameter Name="Timeout">1000</Parameter>
      | 					<Parameter Name="DelayTime">1000000</Parameter>
      | 					<Parameter Name="BufferSize">50</Parameter>
      | 					<Parameter Name="ByteSize">4</Parameter>
      | 					<Parameter Name="CodePage">65001</Parameter>
      | 				</Parameters>
      | 			</SymbolControlItem>
      | 		</SymbolControlItems>
      | 	</Outputs>
      | </PortInfo>
      settings: SourceProductName=Beckhoff TwinCAT Interface
  TwinCAT Sync Clock : TcSimInterface/TwinCAT Sync Clock  ChangeRowColOrder=on  TraceMode=3  DirectFeedThrough=off  SignalLabels=3  PortLabels=2  ExpandBusObjDepth=on  SyncClockMode=Clock  SampleTime=-1
      settings: SourceProductName=Beckhoff TwinCAT Interface
  wires:
  FB_AngleToStroke/2(fKnuckleStroke) -> Simulink-PS Converter/1
  Mux2/1 -> Crane Model (Kinematic)/1(TCP_ref), Scope/1  "TCP_ref"
  FB_JoystickIntegrator/1(fXRef) -> Memory/1, FB_InverceKinematics/1(fXRef), Mux2/1  "xref"
  FB_JoystickIntegrator/2(fYRef) -> Memory1/1, FB_InverceKinematics/2(fYRef), Mux2/2  "yref"
  FB_JoystickIntegrator/3(fZRef) -> Memory2/1, FB_InverceKinematics/3(fZRef), Mux2/3  "zref"
  PS-Simulink Converter5/1 -> FB_InverceKinematics/7(fSlewFeedback)  "slew_angle"
  Constant/1 -> FB_InverceKinematics/6(fZDotRef), FB_InverceKinematics/5(fYDotRef), FB_InverceKinematics/4(fXDotRef)  "vzref"
  FB_StrokeToAngle/2(fKnuckleAngle) -> FB_InverceKinematics/9(fKnuckleFeedback)
  FB_StrokeToAngle/1(fMainAngle) -> FB_InverceKinematics/8(fMainFeedback)
  PS-Simulink Converter4/1 -> FB_StrokeToAngle/1(fMainStroke)  "main_stroke"
  PS-Simulink Converter3/1 -> FB_StrokeToAngle/2(fKnuckleStroke)  "knuckle_stroke"
  FB_InverceKinematics/5(fMainVelRef) -> FB_AngleToStroke/3(fMainAngleVel)
  FB_InverceKinematics/6(fKnuckleVelRef) -> FB_AngleToStroke/4(fKnuckleAngleVel)
  Constant3/1 -> Simulink-PS Converter3/1
  Cast To Double2/1 -> Scope5/3, FB_JoystickIntegrator/3(fJoyZ)
  Constant5/1 -> FB_JoystickIntegrator/4(fCartesianVMax)
  Cast To Double1/1 -> Gain/1
  Constant4/1 -> FB_JoystickIntegrator/5(fTs)
  Tc Symbol Interface1/3 -> Cast To Double2/1  "MAIN.fbCartesianJoystic.fZAxis"
  Cast To Double/1 -> Scope5/1, FB_JoystickIntegrator/1(fJoyX)
  Tc Symbol Interface1/2 -> Cast To Double/1  "MAIN.fbCartesianJoystic.fYAxis"
  Tc Symbol Interface1/1 -> Cast To Double1/1  "MAIN.fbCartesianJoystic.fXAxis"
  FB_AngleToStroke/1(fMainStroke) -> Simulink-PS Converter1/1
  FB_InverceKinematics/7(success) -> Scope3/1
  FB_InverceKinematics/1(fSlewRef) -> Signal_switch/1(slew_false)
  FB_InverceKinematics/2(fMainRef) -> Signal_switch/2(main_false)
  FB_InverceKinematics/3(fKnuckleRef) -> Signal_switch/3(knuckle_false)
  Signal_switch/1(slew_out) -> Simulink-PS Converter2/1
  Signal_switch/2(main_out) -> FB_AngleToStroke/1(fMainAngle)
  Signal_switch/3(knuckle_out) -> FB_AngleToStroke/2(fKnuckleAngle)
  Constant6/1 -> Signal_switch/9(slew_true)
  Constant2/1 -> Signal_switch/8(main_true)
  Constant1/1 -> Signal_switch/7(knuckle_true)
  NOT/1 -> Signal_switch/5(bTrigger)
  Cast To Boolean/1 -> NOT/1
  Step/1 -> Cast To Boolean/1
  Memory/1 -> FB_JoystickIntegrator/6(fXPosFeedBack)
  Memory1/1 -> FB_JoystickIntegrator/7(fYPosFeedBack)
  Memory2/1 -> FB_JoystickIntegrator/8(fZPosFeedBack)
  Gain/1 -> Scope5/2, FB_JoystickIntegrator/2(fJoyY)
  connections:
  Simulink-PS Converter/RConn1 -- Crane Model (Kinematic)/LConn3
  Simulink-PS Converter2/RConn1 -- Crane Model (Kinematic)/LConn1
  Simulink-PS Converter1/RConn1 -- Crane Model (Kinematic)/LConn2
  Simulink-PS Converter3/RConn1 -- Crane Model (Kinematic)/LConn4
  PS-Simulink Converter/LConn1 -- Crane Model (Kinematic)/RConn4
  PS-Simulink Converter1/LConn1 -- Crane Model (Kinematic)/RConn5
  PS-Simulink Converter2/LConn1 -- Crane Model (Kinematic)/RConn6
  PS-Simulink Converter3/LConn1 -- Crane Model (Kinematic)/RConn3
  PS-Simulink Converter4/LConn1 -- Crane Model (Kinematic)/RConn2
  Crane Model (Kinematic)/RConn1 -- PS-Simulink Converter5/LConn1
